simulink model "motor_uart"  (R2025b)
settings: Solver=VariableStepAuto  StartTime=0.0  StopTime=inf  RelTol=1e-3
undefined symbols (not defined in the file or in its folder): CR, LF
libraries: instrumentseriallib x3
settings Model: Creator=diego  LastModifiedBy=diego

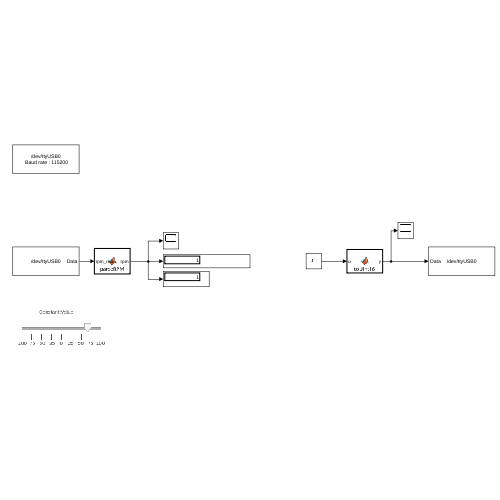
[thumbnail: Simulink's stored preview of the top-level diagram]
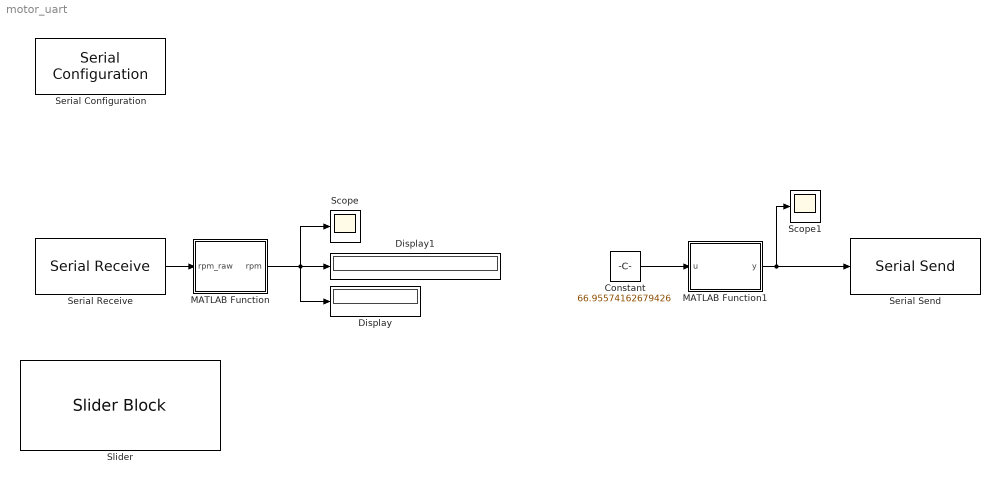
== system motor_uart ==
  Constant : Constant  Value=66.95574162679426
  Display : Display
  Display1 : Display
  MATLAB Function : MATLAB Function  TreatAsAtomicUnit=on
  MATLAB Function1 : MATLAB Function  TreatAsAtomicUnit=on
  Scope : Scope
      settings: ActiveDisplayYMinimum=-82.624999999999986  ActiveDisplayYMaximum=743.625
  Scope1 : Scope
      settings: ActiveDisplayYMinimum=-1  ActiveDisplayYMaximum=1
  Serial Configuration : instrumentseriallib/Serial Configuration  Priority=-200000  PortSel=/dev/ttyUSB0  Port=/dev/ttyUSB0  ComPort=/dev/ttyUSB0  BaudRate=115200  DataBits=8  Parity=none  StopBits=1  ByteOrder=little-endian  FlowControl=none  Timeout=10  SimulateUsing=Interpreted execution  BlockInModel=on  aMode=1
  Serial Receive : instrumentseriallib/Serial Receive  Priority=1  PortSel=/dev/ttyUSB0  Port=/dev/ttyUSB0  ComPort=/dev/ttyUSB0  DataType=int16  SaveDataType=uint8  ToggleHeader=off  Header=[]  ToggleDataSize=on  DataSize=[1 1]  ToggleTerminator=off  Terminator=CR/LF ('\r\n')  CustomTerminator=[]  InputFormat=Column major  EnableBlockingMode=on  ActionDataUnavailable=Output last received value  ActionWhenDataUnavailable=Output last received value  CustomValue=0  SampleTime=0.100  SimulateUsing=Interpreted execution  BlockInModel=on  aMode=1  LibraryInUse=instrumentlib
  Serial Send : instrumentseriallib/Serial Send  Priority=1  PortSel=/dev/ttyUSB0  Port=/dev/ttyUSB0  ComPort=/dev/ttyUSB0  Header=[]  Terminator=<none>  CustomTerminator=[]  EnableBlockingMode=off  SimulateUsing=Interpreted execution  BlockInModel=on  aMode=1
  Slider : SliderBlock  ScaleMin=-100
  wires:
  MATLAB Function/1(rpm) -> Scope/1, Display/1, Display1/1
  Serial Receive/1 -> MATLAB Function/1(rpm_raw)
  Constant/1 -> MATLAB Function1/1(u)
  MATLAB Function1/1(y) -> Scope1/1, Serial Send/1

== matlab function motor_uart/MATLAB Function ==
  data: rpm output; rpm_raw input
function rpm = parseRPM(rpm_raw)
%#codegen
rpm = double(rpm_raw);
end

== matlab function motor_uart/MATLAB Function1 ==
  data: u input; y output
function y = toUint16(u)
v_min = 0;
v_max = 30;

pwm_min = 0;
pwm_max = 65535;

% Escalado lineal
pwm_raw = (u - v_min) * (pwm_max - pwm_min) / (v_max - v_min) + pwm_min;

% Saturación
if pwm_raw > pwm_max * 0.9
    pwm_raw = pwm_max * 0.9;
elseif pwm_raw < pwm_max * 0.1
    pwm_raw = pwm_max * 0.1;
end

% Conversión final
y = uint16(pwm_raw);
end
